simulink model "Suspension_model"  (R2016a)
settings: Solver=ode1  SolverMode=SingleTasking  StartTime=0.0  StopTime=Sim_Time  FixedStep=0.001  RelTol=1e-3
undefined symbols (not defined in the file): A, B, C, D, K
settings Model: Creator=ku53058  LastModifiedBy=Funsho
settings DebuggingCC: SFUnexpectedBacktrackingDiag=error  SFNoUnconditionalDefaultTransitionDiag=error
settings GRTTargetCC: TargetLangStandard=C99 (ISO)  GeneratePreprocessorConditionals=Use local settings
settings ConfigComp: CovMetricSettings=dwe  CovHtmlReporting=off  CovSaveCumulativeToWorkspaceVar=off  CovSaveSingleToWorkspaceVar=off  CovExternalEMLEnable=on

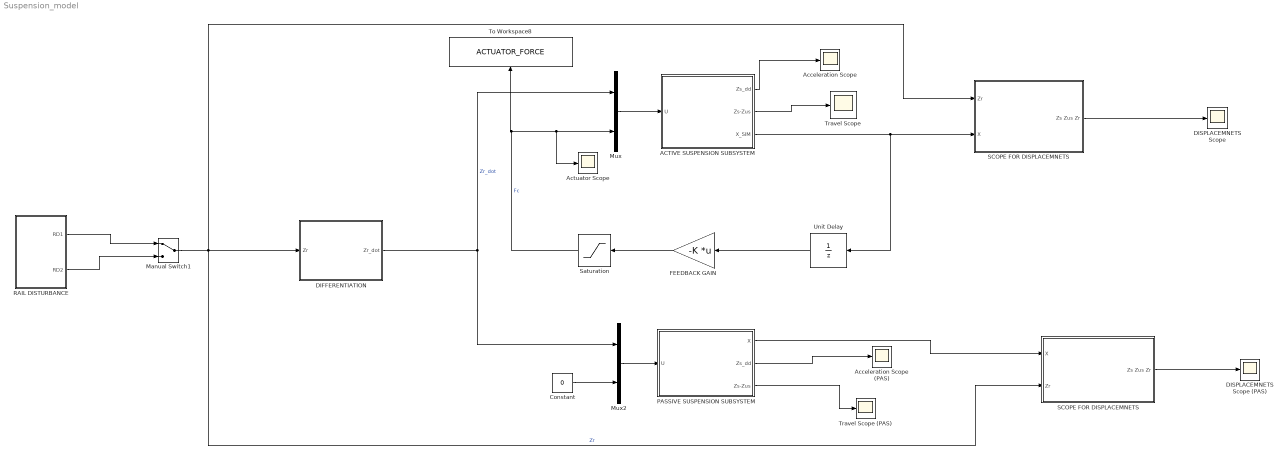
== system Suspension_model ==
  ACTIVE SUSPENSION SUBSYSTEM : Subsystem
  Acceleration Scope : Scope
  Acceleration Scope (PAS) : Scope
  Actuator Scope : Scope
  Constant : Constant  Value=0
  DIFFERENTIATION : Subsystem
  DISPLACEMNETS Scope : Scope
  DISPLACEMNETS Scope (PAS) : Scope
  FEEDBACK GAIN : Gain  Gain=-K  Multiplication=Matrix(K*u)
  Manual Switch1 : ManualSwitch
  Mux : Mux  Inputs=2
  Mux2 : Mux  Inputs=2
  PASSIVE SUSPENSION SUBSYSTEM : Subsystem
  RAIL DISTURBANCE : Subsystem
  SCOPE FOR DISPLACEMNETS : Subsystem
  "SCOPE FOR DISPLACEMNETS " : Subsystem
  Saturation : Saturate  UpperLimit=46730  LowerLimit=-46730
  To Workspace8 : ToWorkspace  VariableName=ACTUATOR_FORCE  SaveFormat=Timeseries  SampleTime=-1
  Travel Scope : Scope
  Travel Scope (PAS) : Scope
  Unit Delay : UnitDelay  SampleTime=-1
  wires:
  FEEDBACK GAIN/1 -> Saturation/1
  Constant/1 -> Mux2/2
  Manual Switch1/1 -> SCOPE FOR DISPLACEMNETS/2(Zr), DIFFERENTIATION/1(Zr), "SCOPE FOR DISPLACEMNETS "/1(Zr)  "Zr"
  Unit Delay/1 -> FEEDBACK GAIN/1
  Saturation/1 -> Mux/2, Actuator Scope/1, To Workspace8/1  "Fc"
  Mux/1 -> ACTIVE SUSPENSION SUBSYSTEM/1(U)
  ACTIVE SUSPENSION SUBSYSTEM/1(Zs_dd) -> Acceleration Scope/1
  ACTIVE SUSPENSION SUBSYSTEM/2(Zs-Zus) -> Travel Scope/1
  ACTIVE SUSPENSION SUBSYSTEM/3(X_SIM) -> Unit Delay/1, "SCOPE FOR DISPLACEMNETS "/2(X)
  "SCOPE FOR DISPLACEMNETS "/1(Zs Zus Zr) -> DISPLACEMNETS Scope/1
  Mux2/1 -> PASSIVE SUSPENSION SUBSYSTEM/1(U)
  PASSIVE SUSPENSION SUBSYSTEM/1(X) -> SCOPE FOR DISPLACEMNETS/1(X)
  SCOPE FOR DISPLACEMNETS/1(Zs Zus Zr) -> DISPLACEMNETS Scope (PAS)/1
  PASSIVE SUSPENSION SUBSYSTEM/2(Zs_dd) -> Acceleration Scope (PAS)/1
  PASSIVE SUSPENSION SUBSYSTEM/3(Zs-Zus) -> Travel Scope (PAS)/1
  RAIL DISTURBANCE/1(RD1) -> Manual Switch1/1
  RAIL DISTURBANCE/2(RD2) -> Manual Switch1/2
  DIFFERENTIATION/1(Zr_dot) -> Mux2/1, Mux/1  "Zr_dot"

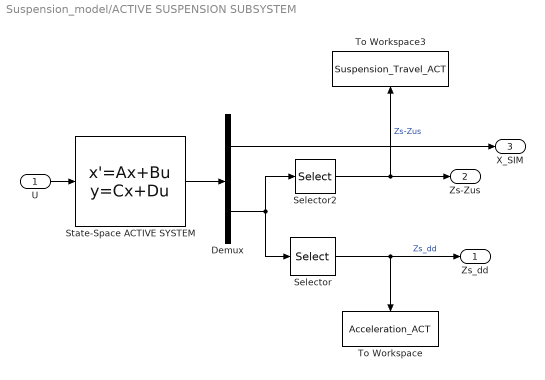
== system Suspension_model/ACTIVE SUSPENSION SUBSYSTEM ==
  U : Inport
  Demux : Demux  Outputs=[4 2]
  Selector : Selector  InputPortWidth=2  IndexOptions=Index vector (dialog)  Indices=[2]  OutputSizes=1
  Selector2 : Selector  InputPortWidth=2  IndexOptions=Index vector (dialog)  Indices=[1]  OutputSizes=1
  State-Space ACTIVE SYSTEM : StateSpace  A=A  B=B  C=cat(1,eye(4), C)  D=D  X0=0
  To Workspace : ToWorkspace  VariableName=Acceleration_ACT  SaveFormat=Timeseries  SampleTime=-1
  To Workspace3 : ToWorkspace  VariableName=Suspension_Travel_ACT  SaveFormat=Timeseries  SampleTime=-1
  Zs_dd : Outport
  Zs-Zus : Outport  Port=2
  X_SIM : Outport  Port=3
  wires:
  Demux/1 -> X_SIM/1
  State-Space ACTIVE SYSTEM/1 -> Demux/1
  Demux/2 -> Selector2/1, Selector/1
  Selector/1 -> Zs_dd/1, To Workspace/1  "Zs_dd"
  Selector2/1 -> Zs-Zus/1, To Workspace3/1  "Zs-Zus"
  U/1 -> State-Space ACTIVE SYSTEM/1

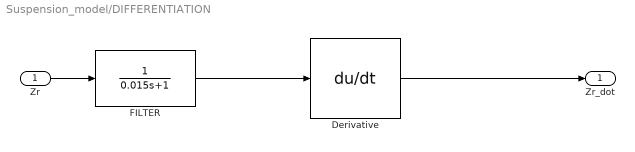
== system Suspension_model/DIFFERENTIATION ==
  Zr : Inport
  Derivative : Derivative
  FILTER : TransferFcn  Denominator=[0.015 1]
  Zr_dot : Outport
  wires:
  FILTER/1 -> Derivative/1
  Derivative/1 -> Zr_dot/1
  Zr/1 -> FILTER/1

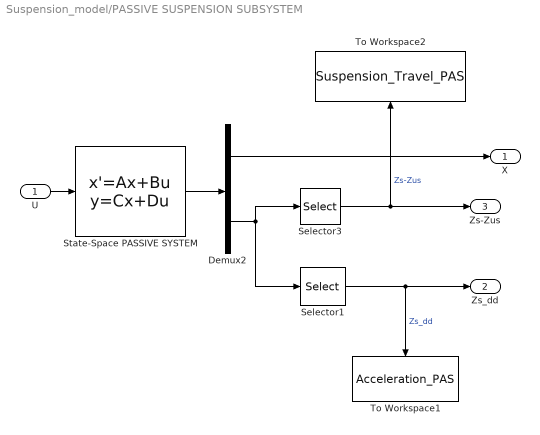
== system Suspension_model/PASSIVE SUSPENSION SUBSYSTEM ==
  U : Inport
  Demux2 : Demux  Outputs=[4 2]
  Selector1 : Selector  InputPortWidth=2  IndexOptions=Index vector (dialog)  Indices=[2]  OutputSizes=1
  Selector3 : Selector  InputPortWidth=2  IndexOptions=Index vector (dialog)  Indices=[1]  OutputSizes=1
  State-Space PASSIVE SYSTEM : StateSpace  A=A  B=B  C=cat(1,eye(4), C)  D=D  X0=0
  To Workspace1 : ToWorkspace  VariableName=Acceleration_PAS  SaveFormat=Timeseries  SampleTime=-1
  To Workspace2 : ToWorkspace  VariableName=Suspension_Travel_PAS  SaveFormat=Timeseries  SampleTime=-1
  X : Outport
  Zs_dd : Outport  Port=2
  Zs-Zus : Outport  Port=3
  wires:
  State-Space PASSIVE SYSTEM/1 -> Demux2/1
  Selector1/1 -> Zs_dd/1, To Workspace1/1  "Zs_dd"
  Demux2/2 -> Selector3/1, Selector1/1
  Selector3/1 -> Zs-Zus/1, To Workspace2/1  "Zs-Zus"
  U/1 -> State-Space PASSIVE SYSTEM/1
  Demux2/1 -> X/1

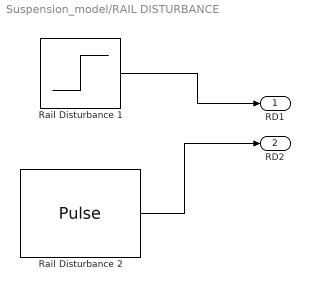
== system Suspension_model/RAIL DISTURBANCE ==
  Rail Disturbance 1 : Step  After=0.06  SampleTime=0
  Rail Disturbance 2 : DiscretePulseGenerator  PulseType=Time based  Amplitude=0.1  Period=6  PulseWidth=50  PhaseDelay=.1
  RD1 : Outport
  RD2 : Outport  Port=2
  wires:
  Rail Disturbance 2/1 -> RD2/1
  Rail Disturbance 1/1 -> RD1/1

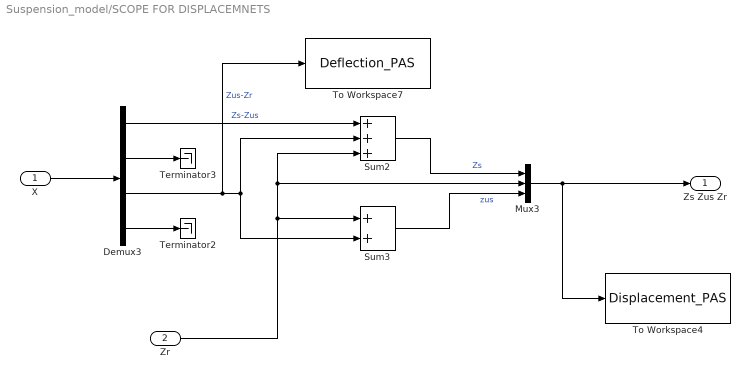
== system Suspension_model/SCOPE FOR DISPLACEMNETS ==
  X : Inport
  Zr : Inport  Port=2
  Demux3 : Demux
  Mux3 : Mux  Inputs=3
  Sum2 : Sum  Inputs=+++
  Sum3 : Sum
  Terminator2 : Terminator
  Terminator3 : Terminator
  To Workspace4 : ToWorkspace  VariableName=Displacement_PAS  SaveFormat=Timeseries  SampleTime=-1
  To Workspace7 : ToWorkspace  VariableName=Deflection_PAS  SaveFormat=Timeseries  SampleTime=-1
  Zs Zus Zr : Outport
  wires:
  Demux3/2 -> Terminator3/1
  Demux3/4 -> Terminator2/1
  Demux3/1 -> Sum2/1  "Zs-Zus"
  Demux3/3 -> To Workspace7/1, Sum3/2, Sum2/2  "Zus-Zr"
  Sum2/1 -> Mux3/1  "Zs"
  Sum3/1 -> Mux3/3  "zus"
  Mux3/1 -> Zs Zus Zr/1, To Workspace4/1
  Zr/1 -> Sum3/1, Mux3/2, Sum2/3
  X/1 -> Demux3/1

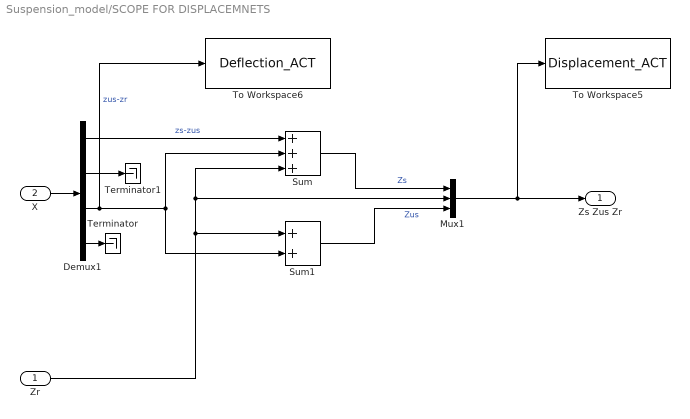
== system Suspension_model/SCOPE FOR DISPLACEMNETS  ==
  Zr : Inport
  X : Inport  Port=2
  Demux1 : Demux
  Mux1 : Mux  Inputs=3
  Sum : Sum  Inputs=+++
  Sum1 : Sum
  Terminator : Terminator
  Terminator1 : Terminator
  To Workspace5 : ToWorkspace  VariableName=Displacement_ACT  SaveFormat=Timeseries  SampleTime=-1
  To Workspace6 : ToWorkspace  VariableName=Deflection_ACT  SaveFormat=Timeseries  SampleTime=-1
  Zs Zus Zr : Outport
  wires:
  X/1 -> Demux1/1
  Demux1/2 -> Terminator1/1
  Demux1/4 -> Terminator/1
  Demux1/1 -> Sum/1  "zs-zus"
  Demux1/3 -> To Workspace6/1, Sum1/2, Sum/2  "zus-zr"
  Sum/1 -> Mux1/1  "Zs"
  Sum1/1 -> Mux1/3  "Zus"
  Mux1/1 -> Zs Zus Zr/1, To Workspace5/1
  Zr/1 -> Sum1/1, Mux1/2, Sum/3
